simulink model "HANcoder_E407_TTA_Controller_v3_2"  (R2018b)
settings: Solver=FixedStepDiscrete  StartTime=0.0  StopTime=1  FixedStep=0.01  RelTol=1e-3
PreLoadFcn:
  | librarySetup
  | eval([bdroot,'_startup']) %Calling [modelName]_startup.m
undefined symbols (not defined in the file): A0, A1, A2, A3, A4, Backup_Board, basic_cycle_duration_bc0, basic_cycle_duration_bc1, comm_delay_estimation1, comm_delay_estimation2, COMM_Period, COMM_Phase1, COMM_Phase2, COMM_Phase_init1, COMM_Phase_init2, COMP_duration, CON2, CON4, Controller1_Board, Controller2_Board, Controller3_Board, D10, D12, D13, D8, D9, delta_a_set, delta_f_set, delta_max, delta_min, delta_precision, e_width, frequency_IRQ, HANtuneOverride, hardware_granularity, I_a, I_f, idle_time_init, Input_Gen_Board, LA_Clock_Gr, LA_COMM_dly, LA_COMM_Err, LA_E_Desync, LA_MEX_Flag, LA_Task_Act, m_v, Master_Role, matrix_cycle_duration, matrix_rows, max_desync, max_num_msgs_CAN1, max_num_msgs_CAN2, min_desync, OutControl1_ID, OutControl2_ID, OutEmulator_ID, R_al, R_ar, R_fl, R_fr ... (+80)
libraries: hdlsllib x434, HANcoder_STM32_Target x28, simulink x3, simulink_extras x1
(part 23 of 31)

== system HANcoder_E407_TTA_Controller_v3_2/HANcoder STM32 Target - E407-STM32 algorithm/TTA CAN System/TTA System/Matrix Cycle Manager/Vehicle Emulator Matrix Cycle/vehicle emulator basic cycle 1/COMM Task - Sync bc 1/Transmission subtasks/Check msg transmission CAN1 ==
  note: The TX buffers are updated one tick
      | before the message is sent
  note: A message should be sent during
      | this tick through CAN1
  note: In the next tick, a message will be
      | sent through CAN1
  Local Time : Inport
  Time Mark : Inport  Port=2
  Tx_ID : Inport  Port=3
  Value Domain Msg : Inport  Port=4
  Enable : EnablePort
  Constant : Constant  Value=COMM_Phase_init1
  Constant11 : Constant  Value=0
  Constant22 : Constant
  Constant24 : Constant  Value=COMM_Phase1
  Constant27 : Constant  Value=COMM_Phase1
  Constant8 : Constant  Value=0
  Equal4 : RelationalOperator  Operator===  OutDataTypeStr=boolean  RndMeth=Simplest
  Equal7 : RelationalOperator  Operator===  OutDataTypeStr=boolean  RndMeth=Simplest
  Minus : Sum  Inputs=++-
  Minus1 : Sum  Inputs=+-
  Minus2 : Sum
  Mod : Math  Operator=mod  SaturateOnIntegerOverflow=on
  Mod1 : Math  Operator=mod  SaturateOnIntegerOverflow=on
  TX buffer update CAN1 : Subsystem  Priority=20
  Send CAN1 : Outport  OutputWhenDisabled=reset  InitialOutput=0
  wires:
  Equal4/1 -> TX buffer update CAN1/Enable
  Constant22/1 -> Minus/2
  Local Time/1 -> Minus1/1, Minus/1
  Tx_ID/1 -> TX buffer update CAN1/1(Tx_ID)
  Mod1/1 -> Equal7/1
  Constant27/1 -> Mod1/2
  Minus/1 -> Mod/1
  Value Domain Msg/1 -> TX buffer update CAN1/2(Msg_Value_Data)
  Constant24/1 -> Mod/2
  Mod/1 -> Equal4/1
  Minus1/1 -> Mod1/1
  Constant11/1 -> Equal7/2
  Equal7/1 -> Send CAN1/1
  Constant8/1 -> Equal4/2
  Constant/1 -> Minus2/2
  Minus2/1 -> Minus1/2, Minus/3
  Time Mark/1 -> Minus2/1

== system HANcoder_E407_TTA_Controller_v3_2/HANcoder STM32 Target - E407-STM32 algorithm/TTA CAN System/TTA System/Matrix Cycle Manager/Vehicle Emulator Matrix Cycle/vehicle emulator basic cycle 1/COMM Task - Sync bc 1/Transmission subtasks/Check msg transmission CAN2 ==
  note: In the next tick, a message will be
      | sent through CAN2
  note: A message should be sent during
      | this tick through CAN2
  note: The TX buffers are updated one tick
      | before the message is sent
  Local Time : Inport
  Time Mark : Inport  Port=2
  Tx_ID : Inport  Port=3
  Value Domain Msg : Inport  Port=4
  Enable : EnablePort
  Constant : Constant  Value=COMM_Phase_init2
  Constant11 : Constant  Value=0
  Constant22 : Constant
  Constant24 : Constant  Value=COMM_Phase2
  Constant27 : Constant  Value=COMM_Phase2
  Constant8 : Constant  Value=0
  Equal4 : RelationalOperator  Operator===  OutDataTypeStr=boolean  RndMeth=Simplest
  Equal7 : RelationalOperator  Operator===  OutDataTypeStr=boolean  RndMeth=Simplest
  Minus : Sum  Inputs=++-
  Minus1 : Sum  Inputs=+-
  Minus2 : Sum
  Mod : Math  Operator=mod  SaturateOnIntegerOverflow=on
  Mod1 : Math  Operator=mod  SaturateOnIntegerOverflow=on
  TX buffer update CAN2 : Subsystem  Priority=20
  Send CAN2 : Outport  OutputWhenDisabled=reset  InitialOutput=0
  wires:
  Constant8/1 -> Equal4/2
  Equal7/1 -> Send CAN2/1
  Constant11/1 -> Equal7/2
  Minus1/1 -> Mod1/1
  Mod/1 -> Equal4/1
  Constant24/1 -> Mod/2
  Value Domain Msg/1 -> TX buffer update CAN2/2(Msg_Value_Data)
  Minus/1 -> Mod/1
  Constant27/1 -> Mod1/2
  Mod1/1 -> Equal7/1
  Tx_ID/1 -> TX buffer update CAN2/1(Tx_ID)
  Local Time/1 -> Minus/1, Minus1/1
  Constant22/1 -> Minus/2
  Equal4/1 -> TX buffer update CAN2/Enable
  Constant/1 -> Minus2/2
  Time Mark/1 -> Minus2/1
  Minus2/1 -> Minus1/2, Minus/3

== system HANcoder_E407_TTA_Controller_v3_2/HANcoder STM32 Target - E407-STM32 algorithm/TTA CAN System/TTA System/Matrix Cycle Manager/Vehicle Emulator Matrix Cycle/vehicle emulator basic cycle 1/COMM Task - Sync bc 1/Transmission subtasks/Msg_Value_Data_Encoded ==
  note: Value domain message encoding
      | <Warning!> The first buffer (from the top) is not used in transmission!
  Enable : EnablePort
  Bus Creator : BusCreator  Inputs=8  OutDataTypeStr=Bus: msg_buffer_type
  Constant : Constant  Value=0  OutDataTypeStr=uint8
  Constant1 : Constant  Value=torque_precision
  Constant10 : Constant  Value=speed_max
  Constant11 : Constant  Value=speed_min
  Constant12 : Constant  Value=delta_max
  Constant13 : Constant  Value=delta_min
  Constant14 : Constant  Value=delta_max
  Constant15 : Constant  Value=delta_min
  Constant2 : Constant  Value=torque_precision
  Constant3 : Constant  Value=speed_precision
  Constant4 : Constant  Value=delta_precision
  Constant5 : Constant  Value=delta_precision
  Constant6 : Constant  Value=tau_max
  Constant7 : Constant  Value=tau_min
  Constant8 : Constant  Value=tau_max
  Constant9 : Constant  Value=tau_min
  Data Store Read33 : DataStoreRead  DataStoreName=speed_integral
  Data Store Read34 : DataStoreRead  DataStoreName=torque_ar_integral
  Data Store Read35 : DataStoreRead  DataStoreName=torque_fr_integral
  Data Store Read36 : DataStoreRead  DataStoreName=delta_a_est
  Data Store Read37 : DataStoreRead  DataStoreName=delta_f_est
  float2uint1 : Subsystem
  float2uint2 : Subsystem
  float2uint3 : Subsystem
  float2uint4 : Subsystem
  float2uint8 : Subsystem
  Value_domain_msg : Outport
  wires:
  Bus Creator/1 -> Value_domain_msg/1
  Constant1/1 -> float2uint8/1(precision)
  Constant2/1 -> float2uint1/1(precision)
  Constant3/1 -> float2uint2/1(precision)
  Constant4/1 -> float2uint3/1(precision)
  Constant5/1 -> float2uint4/1(precision)
  Constant/1 -> Bus Creator/1, Bus Creator/8, Bus Creator/7
  Data Store Read35/1 -> float2uint8/2(magnitude)
  Data Store Read34/1 -> float2uint1/2(magnitude)
  Data Store Read33/1 -> float2uint2/2(magnitude)
  Data Store Read37/1 -> float2uint3/2(magnitude)
  Data Store Read36/1 -> float2uint4/2(magnitude)
  float2uint8/1(coded) -> Bus Creator/2
  float2uint1/1(coded) -> Bus Creator/3
  float2uint2/1(coded) -> Bus Creator/4
  float2uint3/1(coded) -> Bus Creator/5
  float2uint4/1(coded) -> Bus Creator/6
  Constant6/1 -> float2uint8/3(magnitude_max)
  Constant7/1 -> float2uint8/4(magnitude_min)
  Constant9/1 -> float2uint1/4(magnitude_min)
  Constant8/1 -> float2uint1/3(magnitude_max)
  Constant10/1 -> float2uint2/3(magnitude_max)
  Constant11/1 -> float2uint2/4(magnitude_min)
  Constant13/1 -> float2uint3/4(magnitude_min)
  Constant12/1 -> float2uint3/3(magnitude_max)
  Constant14/1 -> float2uint4/3(magnitude_max)
  Constant15/1 -> float2uint4/4(magnitude_min)

== system HANcoder_E407_TTA_Controller_v3_2/HANcoder STM32 Target - E407-STM32 algorithm/TTA CAN System/TTA System/Matrix Cycle Manager/Vehicle Emulator Matrix Cycle/vehicle emulator basic cycle 1/COMP Task - Rx Output Emulator Check/Process_Messages/Demux message CAN1 and check coherence ==
  CAN1_Rx_msg : Inport  OutDataTypeStr=Bus: msg_buffer_type
  expected_board_id : Inport  Port=2
  Enable : EnablePort
  Bus Creator : BusCreator  Inputs=8  OutDataTypeStr=Bus: msg_buffer_type
  Bus Selector : BusSelector  OutputSignals=Buffer_1,Buffer_2,Buffer_3,Buffer_4,Buffer_5,Buffer_6,Buffer_7,Buffer_8
  Constant : Constant  Value=0  OutDataTypeStr=uint8
  Equal : RelationalOperator  Operator===  OutDataTypeStr=boolean  RndMeth=Simplest
  Subsystem : Subsystem
  Terminator : Terminator
  msg_count>2_DEBUG : Subsystem
  CAN1_msg : Outport  OutDataTypeStr=Bus: msg_buffer_type
  Msg_Count_CAN1 : Outport  Port=2
  CAN1_msg_coherent : Outport  Port=3  OutputWhenDisabled=reset  InitialOutput=0
  wires:
  Bus Selector/2 -> Bus Creator/2  "<Buffer_2>"
  Bus Selector/3 -> Bus Creator/3  "<Buffer_3>"
  CAN1_Rx_msg/1 -> Bus Selector/1
  Equal/1 -> CAN1_msg_coherent/1
  expected_board_id/1 -> Equal/2
  Bus Selector/6 -> Bus Creator/6  "<Buffer_6>"
  Bus Selector/5 -> Bus Creator/5  "<Buffer_5>"
  Bus Selector/7 -> Bus Creator/7  "<Buffer_7>"
  Bus Selector/8 -> Bus Creator/8  "<Buffer_8>"
  Bus Selector/4 -> Bus Creator/4  "<Buffer_4>"
  Subsystem/3(board_id) -> Equal/1
  Bus Selector/1 -> Subsystem/1(Msg_Temporal_Data)  "<Buffer_1>"
  Subsystem/2(msg_count) -> msg_count>2_DEBUG/1(msg_c), Msg_Count_CAN1/1
  Bus Creator/1 -> CAN1_msg/1
  Constant/1 -> Bus Creator/1
  Subsystem/1(basic_cycle) -> Terminator/1

== system HANcoder_E407_TTA_Controller_v3_2/HANcoder STM32 Target - E407-STM32 algorithm/TTA CAN System/TTA System/Matrix Cycle Manager/Vehicle Emulator Matrix Cycle/vehicle emulator basic cycle 1/COMP Task - Rx Output Emulator Check/Process_Messages/Demux message CAN1 and check coherence1 ==
  CAN2_Rx_msg : Inport  OutDataTypeStr=Bus: msg_buffer_type
  expected_board_id : Inport  Port=2
  Enable : EnablePort
  Bus Creator : BusCreator  Inputs=8  OutDataTypeStr=Bus: msg_buffer_type
  Bus Selector : BusSelector  OutputSignals=Buffer_1,Buffer_2,Buffer_3,Buffer_4,Buffer_5,Buffer_6,Buffer_7,Buffer_8
  Constant : Constant  Value=0  OutDataTypeStr=uint8
  Equal : RelationalOperator  Operator===  OutDataTypeStr=boolean  RndMeth=Simplest
  Subsystem : Subsystem
  Terminator : Terminator
  msg_count>2_DEBUG : Subsystem
  CAN2_msg_coherent : Outport  OutputWhenDisabled=reset  InitialOutput=0
  Msg_Count_CAN2 : Outport  Port=2
  CAN2_msg : Outport  Port=3  OutDataTypeStr=Bus: msg_buffer_type
  wires:
  Bus Selector/2 -> Bus Creator/2  "<Buffer_2>"
  Bus Selector/3 -> Bus Creator/3  "<Buffer_3>"
  CAN2_Rx_msg/1 -> Bus Selector/1
  Equal/1 -> CAN2_msg_coherent/1
  expected_board_id/1 -> Equal/2
  Bus Selector/6 -> Bus Creator/6  "<Buffer_6>"
  Bus Selector/5 -> Bus Creator/5  "<Buffer_5>"
  Bus Selector/7 -> Bus Creator/7  "<Buffer_7>"
  Bus Selector/8 -> Bus Creator/8  "<Buffer_8>"
  Bus Selector/4 -> Bus Creator/4  "<Buffer_4>"
  Subsystem/3(board_id) -> Equal/1
  Bus Selector/1 -> Subsystem/1(Msg_Temporal_Data)  "<Buffer_1>"
  Subsystem/2(msg_count) -> msg_count>2_DEBUG/1(msg_c), Msg_Count_CAN2/1
  Bus Creator/1 -> CAN2_msg/1
  Constant/1 -> Bus Creator/1
  Subsystem/1(basic_cycle) -> Terminator/1

== system HANcoder_E407_TTA_Controller_v3_2/HANcoder STM32 Target - E407-STM32 algorithm/TTA CAN System/TTA System/Matrix Cycle Manager/Vehicle Emulator Matrix Cycle/vehicle emulator basic cycle 1/COMP Task - Rx Output Emulator Check/Update Msg buffer/Sensor Values Rx Update ==
  note: If we miss any msg, with current version we
      | suppose vehicle emulator remains in the same
      | state until new msg is received.
  note: Reinitialize variables
  note: Ticks to seconds conversion
  note: Matrix cycles since last input value
  note: For derivatives and integrals it is important to keep
      | track of how much time has passed since the last
      | time we received a controller value.
  msg_rx : Inport
  Enable : EnablePort
  Bus Selector : BusSelector  OutputSignals=Buffer_2,Buffer_3,Buffer_4,Buffer_5
  Constant : Constant  Value=matrix_cycle_duration
  Constant{1..4} (4 alike) : Constant  Value=torque_precision
  Constant5 : Constant
  Constant6 : Constant  Value=0  OutDataTypeStr=boolean
  Constant7 : Constant
  Data Store Read1 : DataStoreRead  DataStoreName=mc_counter
  Data Store Write : DataStoreWrite  DataStoreName=torque_fr
  Data Store Write1 : DataStoreWrite  DataStoreName=torque_fl
  Data Store Write2 : DataStoreWrite  DataStoreName=torque_ar
  Data Store Write3 : DataStoreWrite  DataStoreName=torque_al
  Data Store Write4 : DataStoreWrite  Priority=1  DataStoreName=rx_data_incr_time
  Data Store Write5 : DataStoreWrite  Priority=2  DataStoreName=mc_counter
  Data Store Write6 : DataStoreWrite  DataStoreName=controller_msg_missed
  Gain : Gain  Gain=frequency_IRQ/hardware_granularity
  Multiply : Product
  Terminator : Terminator
  uint8_2float : Subsystem
  uint8_2float1 : Subsystem
  uint8_2float2 : Subsystem
  uint8_2float3 : Subsystem
  wires:
  msg_rx/1 -> Bus Selector/1
  Bus Selector/3 -> uint8_2float2/2(value)  "<Buffer_4>"
  Bus Selector/2 -> uint8_2float1/2(value)  "<Buffer_3>"
  Bus Selector/1 -> uint8_2float/2(value)  "<Buffer_2>"
  Bus Selector/4 -> uint8_2float3/2(value)  "<Buffer_5>"
  Constant4/1 -> uint8_2float/1(precision)
  Constant1/1 -> uint8_2float1/1(precision)
  Constant2/1 -> uint8_2float2/1(precision)
  Constant3/1 -> uint8_2float3/1(precision)
  uint8_2float3/1(decoded) -> Data Store Write3/1
  uint8_2float2/1(decoded) -> Data Store Write2/1
  uint8_2float1/1(decoded) -> Data Store Write1/1
  uint8_2float/1(decoded) -> Data Store Write/1
  Constant5/1 -> Data Store Write5/1
  Gain/1 -> Multiply/1
  Constant7/1 -> Multiply/2
  Multiply/1 -> Data Store Write4/1
  Constant/1 -> Gain/1
  Constant6/1 -> Data Store Write6/1
  Data Store Read1/1 -> Terminator/1

== system HANcoder_E407_TTA_Controller_v3_2/HANcoder STM32 Target - E407-STM32 algorithm/TTA CAN System/TTA System/Matrix Cycle Manager/Vehicle Emulator Matrix Cycle/vehicle emulator basic cycle 1/COMP Task - Rx Output Emulator Check/Update Msg buffer/Sensor Values not Rx Update ==
  note: If no inputs received, no calculations are done.
      | Next time controller values are received
      | it is important to keep track of how much time
      | has passed for derivatives and integrals.
  Enable : EnablePort
  Constant1 : Constant
  Constant2 : Constant  OutDataTypeStr=boolean
  Data Store Read : DataStoreRead  DataStoreName=mc_counter
  Data Store Write : DataStoreWrite  DataStoreName=controller_msg_missed
  Data Store Write1 : DataStoreWrite  DataStoreName=mc_counter
  Minus : Sum
  wires:
  Minus/1 -> Data Store Write1/1
  Constant1/1 -> Minus/2
  Data Store Read/1 -> Minus/1
  Constant2/1 -> Data Store Write/1

== system HANcoder_E407_TTA_Controller_v3_2/HANcoder STM32 Target - E407-STM32 algorithm/TTA CAN System/TTA System/Matrix Cycle Manager/Vehicle Emulator Matrix Cycle/vehicle emulator basic cycle 1/COMP Task - Sync bc1 check/Process_Messages/Demux message CAN1 and check coherence ==
  CAN1_Rx_msg : Inport  OutDataTypeStr=Bus: msg_buffer_type
  expected_basic_cycle : Inport  Port=2
  Enable : EnablePort
  Bus Creator : BusCreator  Inputs=8  OutDataTypeStr=Bus: msg_buffer_type
  Bus Selector : BusSelector  OutputSignals=Buffer_1,Buffer_2,Buffer_3,Buffer_4,Buffer_5,Buffer_6,Buffer_7,Buffer_8
  Constant : Constant  Value=0  OutDataTypeStr=uint8
  Equal1 : RelationalOperator  Operator===  OutDataTypeStr=boolean  RndMeth=Simplest
  Subsystem : Subsystem
  Terminator : Terminator
  msg_count>2_DEBUG : Subsystem
  CAN1_msg : Outport  OutDataTypeStr=Bus: msg_buffer_type
  Msg_Count_CAN1 : Outport  Port=2
  CAN1_msg_coherent : Outport  Port=3  OutputWhenDisabled=reset  InitialOutput=0
  wires:
  Bus Selector/2 -> Bus Creator/2  "<Buffer_2>"
  Bus Selector/3 -> Bus Creator/3  "<Buffer_3>"
  CAN1_Rx_msg/1 -> Bus Selector/1
  Equal1/1 -> CAN1_msg_coherent/1
  expected_basic_cycle/1 -> Equal1/2
  Bus Selector/6 -> Bus Creator/6  "<Buffer_6>"
  Bus Selector/5 -> Bus Creator/5  "<Buffer_5>"
  Bus Selector/7 -> Bus Creator/7  "<Buffer_7>"
  Bus Selector/8 -> Bus Creator/8  "<Buffer_8>"
  Bus Selector/4 -> Bus Creator/4  "<Buffer_4>"
  Bus Selector/1 -> Subsystem/1(Msg_Temporal_Data)  "<Buffer_1>"
  Subsystem/1(basic_cycle) -> Equal1/1
  Subsystem/2(msg_count) -> msg_count>2_DEBUG/1(msg_c), Msg_Count_CAN1/1
  Bus Creator/1 -> CAN1_msg/1
  Constant/1 -> Bus Creator/1
  Subsystem/3(board_id) -> Terminator/1

== system HANcoder_E407_TTA_Controller_v3_2/HANcoder STM32 Target - E407-STM32 algorithm/TTA CAN System/TTA System/Matrix Cycle Manager/Vehicle Emulator Matrix Cycle/vehicle emulator basic cycle 1/COMP Task - Sync bc1 check/Process_Messages/Demux message CAN1 and check coherence1 ==
  CAN2_Rx_msg : Inport  OutDataTypeStr=Bus: msg_buffer_type
  expected_basic_cycle : Inport  Port=2
  Enable : EnablePort
  Bus Creator : BusCreator  Inputs=8  OutDataTypeStr=Bus: msg_buffer_type
  Bus Selector : BusSelector  OutputSignals=Buffer_1,Buffer_2,Buffer_3,Buffer_4,Buffer_5,Buffer_6,Buffer_7,Buffer_8
  Constant : Constant  Value=0  OutDataTypeStr=uint8
  Equal1 : RelationalOperator  Operator===  OutDataTypeStr=boolean  RndMeth=Simplest
  Subsystem : Subsystem
  Terminator : Terminator
  msg_count>2_DEBUG : Subsystem
  CAN2_msg_coherent : Outport  OutputWhenDisabled=reset  InitialOutput=0
  Msg_Count_CAN2 : Outport  Port=2
  CAN2_msg : Outport  Port=3  OutDataTypeStr=Bus: msg_buffer_type
  wires:
  Bus Selector/2 -> Bus Creator/2  "<Buffer_2>"
  Bus Selector/3 -> Bus Creator/3  "<Buffer_3>"
  CAN2_Rx_msg/1 -> Bus Selector/1
  Equal1/1 -> CAN2_msg_coherent/1
  expected_basic_cycle/1 -> Equal1/2
  Bus Selector/6 -> Bus Creator/6  "<Buffer_6>"
  Bus Selector/5 -> Bus Creator/5  "<Buffer_5>"
  Bus Selector/7 -> Bus Creator/7  "<Buffer_7>"
  Bus Selector/8 -> Bus Creator/8  "<Buffer_8>"
  Bus Selector/4 -> Bus Creator/4  "<Buffer_4>"
  Bus Selector/1 -> Subsystem/1(Msg_Temporal_Data)  "<Buffer_1>"
  Subsystem/1(basic_cycle) -> Equal1/1
  Subsystem/2(msg_count) -> Msg_Count_CAN2/1, msg_count>2_DEBUG/1(msg_c)
  Bus Creator/1 -> CAN2_msg/1
  Constant/1 -> Bus Creator/1
  Subsystem/3(board_id) -> Terminator/1

== system HANcoder_E407_TTA_Controller_v3_2/HANcoder STM32 Target - E407-STM32 algorithm/TTA CAN System/TTA System/Matrix Cycle Manager/Vehicle Emulator Matrix Cycle/vehicle emulator basic cycle 1/COMP Task - Sync bc1 check/Process_Messages/Desync calculation ==
  note: Estimation of the Local Time when the message was sent
  note: Desync CAN2
      | expected RX - Actual RX
  note: Desync CAN1
      | expected RX - Actual RX
  TM_COMM : Inport
  New_msg_CAN1 : Inport  Port=2
  msg_count_CAN1 : Inport  Port=3
  msg_count_CAN2 : Inport  Port=4
  Enable : EnablePort
  Constant : Constant  Value=COMM_Phase1
  Constant1 : Constant  Value=COMM_Phase2
  Data Store Read : DataStoreRead  DataStoreName=Msg_Rx_Ticks_CAN1
  Data Store Read1 : DataStoreRead  DataStoreName=Msg_Rx_Ticks_CAN2
  Data Store Write1 : DataStoreWrite  Priority=23  DataStoreName=Desync_Ticks
  Minus : Sum  Priority=21  Inputs=+-
  Minus1 : Sum  Priority=20  Inputs=+-
  Multiply : Product  Priority=10
  Multiply1 : Product  Priority=12
  Saturation : Saturate  UpperLimit=max_desync  LowerLimit=min_desync
  Sum : Sum  Priority=11  Inputs=+++
  Sum1 : Sum  Priority=13  Inputs=+++
  Switch1 : Switch  Priority=22  Criteria=u2 > Threshold
  delay_estimation_1 : Constant  Value=comm_delay_estimation1
  delay_estimation_2 : Constant  Value=comm_delay_estimation2
  wires:
  TM_COMM/1 -> Sum1/2, Sum/2
  delay_estimation_1/1 -> Sum/3
  msg_count_CAN1/1 -> Multiply/2
  Switch1/1 -> Saturation/1
  Minus/1 -> Switch1/3
  Sum1/1 -> [expected_LT_CAN2]
  delay_estimation_2/1 -> Sum1/3
  Multiply1/1 -> Sum1/1
  [expected_LT_CAN1] -> Minus1/1
  [expected_LT_CAN2] -> Minus/1
  Data Store Read1/1 -> Minus/2
  Multiply/1 -> Sum/1
  Data Store Read/1 -> Minus1/2
  msg_count_CAN2/1 -> Multiply1/2
  Sum/1 -> [expected_LT_CAN1]
  Minus1/1 -> Switch1/1
  Constant/1 -> Multiply/1
  Constant1/1 -> Multiply1/1
  New_msg_CAN1/1 -> Switch1/2
  Saturation/1 -> Data Store Write1/1  "Desync_Sync_bc1_vem_s"

== system HANcoder_E407_TTA_Controller_v3_2/HANcoder STM32 Target - E407-STM32 algorithm/TTA CAN System/TTA System/Matrix Cycle Manager/Vehicle Emulator Matrix Cycle/vehicle emulator basic cycle 1/COMP Task - Update LT/Local Time Update/Desync_Negative ==
  note: Local Time Update
  note: Current Local Time correction
  note: Local time correction when Desync is negative
      | In this case the Local Time "goes back in time".
      | Previous tasks will not be activated because
      | sync_processed flag is alread set.
  Current_Local_Time : Inport
  Enable : EnablePort
  Cast : DataTypeConversion  Priority=13  OutDataTypeStr=uint16
  Data Store Read : DataStoreRead  Priority=11  DataStoreName=Desync_Ticks
  Data Store Write1 : DataStoreWrite  Priority=14  DataStoreName=Local_Ticks  DataStoreElements=Local_Ticks
  Minus : Sum  Priority=12
  wires:
  Current_Local_Time/1 -> Minus/1
  Cast/1 -> Data Store Write1/1
  Minus/1 -> Cast/1
  Data Store Read/1 -> Minus/2

== system HANcoder_E407_TTA_Controller_v3_2/HANcoder STM32 Target - E407-STM32 algorithm/TTA CAN System/TTA System/Matrix Cycle Manager/Backup Board Matrix Cycle/Backup board basic cycle 0/COMM Task - Sync bc 0/Transmission subtasks/Check msg transmission CAN1/TX buffer update CAN1 ==
  note: Transmission end - Set message to send through CAN 1
  note: Message Temporal Data
      |    Every message sends
      |    BasicCycle, Tx count
      |    and Verification msg
      |    as data
  note: Transmission ID
      |    Sync Msg: 1
      |    Vote Node 1: 11
      |    Vote Node 2: 12
      |    Vote Node 3: 13
  Tx_ID : Inport
  Msg_Value_Data : Inport  Port=2
  Enable : EnablePort
  Bus Selector : BusSelector  OutputSignals=signal2,signal3,signal4,signal5,signal6,signal7,signal8
  Cast : DataTypeConversion  OutDataTypeStr=uint32
  Cast1 : DataTypeConversion  OutDataTypeStr=uint8
  Cast16 : DataTypeConversion  OutDataTypeStr=uint8
  Cast4 : DataTypeConversion  OutDataTypeStr=uint8
  Data Store Read : DataStoreRead  Priority=50  DataStoreName=Tx_msg_count_CAN1
  Data Store Read1 : DataStoreRead  DataStoreName=Board_ID
  Data Store Read3 : DataStoreRead  DataStoreName=basic_cycle_count
  Data Store Write10 : DataStoreWrite  DataStoreName=Msg_Tx_CAN1  DataStoreElements=Msg_Tx_CAN1.Buffer_1#Msg_Tx_CAN1.Buffer_2#Msg_Tx_CAN1.Buffer_3#Msg_Tx_CAN1.Buffer_4#Msg_Tx_CAN1.Buffer_5#Msg_Tx_CAN1.Buffer_6#Msg_Tx_CAN1.Buffer_7#Msg_Tx_CAN1.Buffer_8
  Data Store Write8 : DataStoreWrite  DataStoreName=TxID_CAN1
  Msg_Data_Encoder : Subsystem
  wires:
  Cast/1 -> Data Store Write8/1
  Data Store Read3/1 -> Cast4/1
  Cast4/1 -> Msg_Data_Encoder/1(basic_cycle)
  Msg_Value_Data/1 -> Bus Selector/1
  Tx_ID/1 -> Cast/1
  Data Store Read/1 -> Cast1/1
  Cast16/1 -> Msg_Data_Encoder/3(board_number)
  Cast1/1 -> Msg_Data_Encoder/2(tx_counter)
  Data Store Read1/1 -> Cast16/1
  Msg_Data_Encoder/1(encoded_msg) -> Data Store Write10/1
  Bus Selector/1 -> Data Store Write10/2  "<signal2>"
  Bus Selector/2 -> Data Store Write10/3  "<signal3>"
  Bus Selector/3 -> Data Store Write10/4  "<signal4>"
  Bus Selector/4 -> Data Store Write10/5  "<signal5>"
  Bus Selector/5 -> Data Store Write10/6  "<signal6>"
  Bus Selector/6 -> Data Store Write10/7  "<signal7>"
  Bus Selector/7 -> Data Store Write10/8  "<signal8>"

== system HANcoder_E407_TTA_Controller_v3_2/HANcoder STM32 Target - E407-STM32 algorithm/TTA CAN System/TTA System/Matrix Cycle Manager/Backup Board Matrix Cycle/Backup board basic cycle 0/COMM Task - Sync bc 0/Transmission subtasks/Check msg transmission CAN2/TX buffer update CAN2 ==
  note: Transmission end - Set message to send through CAN
  note: Transmission ID
      |    Sync Msg: 1
      |    Vote Node 1: 11
      |    Vote Node 2: 12
      |    Vote Node 3: 13
  note: Message Data
      |    Every message sends
      |    BasicCycle, Tx count
      |    and Verification msg
      |    as data
  Tx_ID : Inport
  Msg_Value_Data : Inport  Port=2
  Enable : EnablePort
  Bus Selector : BusSelector  OutputSignals=signal2,signal3,signal4,signal5,signal6,signal7,signal8
  Cast17 : DataTypeConversion  OutDataTypeStr=uint8
  Cast18 : DataTypeConversion  OutDataTypeStr=uint8
  Cast8 : DataTypeConversion  OutDataTypeStr=uint32
  Cast9 : DataTypeConversion  OutDataTypeStr=uint8
  Data Store Read : DataStoreRead  DataStoreName=Board_ID
  Data Store Read1 : DataStoreRead  Priority=50  DataStoreName=Tx_msg_count_CAN2
  Data Store Read6 : DataStoreRead  DataStoreName=basic_cycle_count
  Data Store Write4 : DataStoreWrite  DataStoreName=Msg_Tx_CAN2  DataStoreElements=Msg_Tx_CAN2.Buffer_1#Msg_Tx_CAN2.Buffer_2#Msg_Tx_CAN2.Buffer_3#Msg_Tx_CAN2.Buffer_4#Msg_Tx_CAN2.Buffer_5#Msg_Tx_CAN2.Buffer_6#Msg_Tx_CAN2.Buffer_7#Msg_Tx_CAN2.Buffer_8
  Data Store Write5 : DataStoreWrite  DataStoreName=TxID_CAN2
  Msg_Data_Encoder : Subsystem
  wires:
  Bus Selector/7 -> Data Store Write4/8  "<signal8>"
  Bus Selector/6 -> Data Store Write4/7  "<signal7>"
  Bus Selector/5 -> Data Store Write4/6  "<signal6>"
  Bus Selector/4 -> Data Store Write4/5  "<signal5>"
  Bus Selector/3 -> Data Store Write4/4  "<signal4>"
  Bus Selector/2 -> Data Store Write4/3  "<signal3>"
  Bus Selector/1 -> Data Store Write4/2  "<signal2>"
  Msg_Value_Data/1 -> Bus Selector/1
  Data Store Read/1 -> Cast17/1
  Cast8/1 -> Data Store Write5/1
  Cast9/1 -> Msg_Data_Encoder/2(tx_counter)
  Tx_ID/1 -> Cast8/1
  Cast17/1 -> Msg_Data_Encoder/3(verif_value)
  Data Store Read6/1 -> Cast18/1
  Msg_Data_Encoder/1(encoded_msg) -> Data Store Write4/1
  Data Store Read1/1 -> Cast9/1
  Cast18/1 -> Msg_Data_Encoder/1(basic_cycle)

== system HANcoder_E407_TTA_Controller_v3_2/HANcoder STM32 Target - E407-STM32 algorithm/TTA CAN System/TTA System/Matrix Cycle Manager/Backup Board Matrix Cycle/Backup board basic cycle 0/COMM Task - Sync bc 0/Transmission subtasks/Msg_Value_Data_Encoded/float2uint1 ==
  precision : Inport
  magnitude : Inport  Port=2
  magnitude_max : Inport  Port=3
  magnitude_min : Inport  Port=4
  Abs : Abs
  Bit Shift : hdlsllib/Logic and Bit Operations/Bit Shift  mode=Shift Left Logical  N=7
      settings: SourceProductName=HDL Coder  SourceProductBaseCode=HD
  Cast : DataTypeConversion  OutDataTypeStr=uint8
  Cast1 : DataTypeConversion  OutDataTypeStr=uint8
  Cast2 : DataTypeConversion  OutDataTypeStr=uint8
  Constant : Constant  Value=0
  Constant1 : Constant  Value=2
  Constant2 : Constant  Value=2
  Divide : Product  Inputs=*/
  Fix : Rounding  Priority=3  Operator=fix
  Fix1 : Rounding  Priority=6  Operator=fix
  Gain : Gain  Gain=-1
  GreaterThan : RelationalOperator  Priority=2  Operator=<  OutDataTypeStr=boolean  RndMeth=Simplest
  LessThanOrEqual1 : RelationalOperator  OutDataTypeStr=boolean  RndMeth=Simplest
  LessThanOrEqual2 : RelationalOperator  Operator=<  OutDataTypeStr=boolean  RndMeth=Simplest
  Minus : Sum  Priority=4  Inputs=-+
  Multiply : Product
  Plus : Sum  Priority=10  Inputs=+++
  Power : Math  Priority=5  Operator=pow  SaturateOnIntegerOverflow=on
  Power1 : Math  Priority=5  Operator=pow  SaturateOnIntegerOverflow=on
  Switch : Switch  Criteria=u2 > Threshold
  Switch1 : Switch  Criteria=u2 > Threshold
  Switch2 : Switch  Criteria=u2 > Threshold
  coded : Outport
  wires:
  Switch1/1 -> Switch2/3
  Switch/1 -> Switch2/1
  LessThanOrEqual1/1 -> Switch1/2
  LessThanOrEqual2/1 -> Switch/2, Switch2/2
  magnitude_max/1 -> LessThanOrEqual2/1, Switch/1
  magnitude_min/1 -> Switch1/3, LessThanOrEqual1/2
  magnitude/1 -> Switch/3, LessThanOrEqual2/2, Switch1/1, LessThanOrEqual1/1
  Plus/1 -> coded/1
  [prec] -> Power1/2
  Multiply/1 -> Cast1/1
  precision/1 -> Gain/1, [prec]
  Power1/1 -> Multiply/2
  Constant2/1 -> Power1/1
  Cast2/1 -> Plus/3
  Fix1/1 -> Cast2/1
  Divide/1 -> Fix1/1
  Power/1 -> Divide/2
  Gain/1 -> Power/2
  Constant1/1 -> Power/1
  Cast1/1 -> Plus/2
  Bit Shift/1 -> Plus/1
  Cast/1 -> Bit Shift/1
  Minus/1 -> Divide/1
  Fix/1 -> Minus/1, Multiply/1
  GreaterThan/1 -> Cast/1
  Abs/1 -> Fix/1, Minus/2
  Switch2/1 -> GreaterThan/1, Abs/1
  Constant/1 -> GreaterThan/2

== system HANcoder_E407_TTA_Controller_v3_2/HANcoder STM32 Target - E407-STM32 algorithm/TTA CAN System/TTA System/Matrix Cycle Manager/Backup Board Matrix Cycle/Backup board basic cycle 0/COMM Task - Sync bc 0/Transmission subtasks/Msg_Value_Data_Encoded/float2uint2 ==
  precision : Inport
  magnitude : Inport  Port=2
  magnitude_max : Inport  Port=3
  magnitude_min : Inport  Port=4
  Abs : Abs
  Bit Shift : hdlsllib/Logic and Bit Operations/Bit Shift  mode=Shift Left Logical  N=7
      settings: SourceProductName=HDL Coder  SourceProductBaseCode=HD
  Cast : DataTypeConversion  OutDataTypeStr=uint8
  Cast1 : DataTypeConversion  OutDataTypeStr=uint8
  Cast2 : DataTypeConversion  OutDataTypeStr=uint8
  Constant : Constant  Value=0
  Constant1 : Constant  Value=2
  Constant2 : Constant  Value=2
  Divide : Product  Inputs=*/
  Fix : Rounding  Priority=3  Operator=fix
  Fix1 : Rounding  Priority=6  Operator=fix
  Gain : Gain  Gain=-1
  GreaterThan : RelationalOperator  Priority=2  Operator=<  OutDataTypeStr=boolean  RndMeth=Simplest
  LessThanOrEqual1 : RelationalOperator  OutDataTypeStr=boolean  RndMeth=Simplest
  LessThanOrEqual2 : RelationalOperator  Operator=<  OutDataTypeStr=boolean  RndMeth=Simplest
  Minus : Sum  Priority=4  Inputs=-+
  Multiply : Product
  Plus : Sum  Priority=10  Inputs=+++
  Power : Math  Priority=5  Operator=pow  SaturateOnIntegerOverflow=on
  Power1 : Math  Priority=5  Operator=pow  SaturateOnIntegerOverflow=on
  Switch : Switch  Criteria=u2 > Threshold
  Switch1 : Switch  Criteria=u2 > Threshold
  Switch2 : Switch  Criteria=u2 > Threshold
  coded : Outport
  wires:
  Constant/1 -> GreaterThan/2
  Switch2/1 -> Abs/1, GreaterThan/1
  Abs/1 -> Minus/2, Fix/1
  GreaterThan/1 -> Cast/1
  Fix/1 -> Multiply/1, Minus/1
  Minus/1 -> Divide/1
  Cast/1 -> Bit Shift/1
  Bit Shift/1 -> Plus/1
  Cast1/1 -> Plus/2
  Constant1/1 -> Power/1
  Gain/1 -> Power/2
  Power/1 -> Divide/2
  Divide/1 -> Fix1/1
  Fix1/1 -> Cast2/1
  Cast2/1 -> Plus/3
  Constant2/1 -> Power1/1
  Power1/1 -> Multiply/2
  precision/1 -> [prec], Gain/1
  Multiply/1 -> Cast1/1
  [prec] -> Power1/2
  Plus/1 -> coded/1
  magnitude/1 -> LessThanOrEqual1/1, Switch1/1, LessThanOrEqual2/2, Switch/3
  magnitude_min/1 -> LessThanOrEqual1/2, Switch1/3
  magnitude_max/1 -> Switch/1, LessThanOrEqual2/1
  LessThanOrEqual2/1 -> Switch2/2, Switch/2
  LessThanOrEqual1/1 -> Switch1/2
  Switch/1 -> Switch2/1
  Switch1/1 -> Switch2/3

== system HANcoder_E407_TTA_Controller_v3_2/HANcoder STM32 Target - E407-STM32 algorithm/TTA CAN System/TTA System/Matrix Cycle Manager/Backup Board Matrix Cycle/Backup board basic cycle 0/COMM Task - Sync bc 0/Transmission subtasks/Msg_Value_Data_Encoded/float2uint3 ==
  precision : Inport
  magnitude : Inport  Port=2
  magnitude_max : Inport  Port=3
  magnitude_min : Inport  Port=4
  Abs : Abs
  Bit Shift : hdlsllib/Logic and Bit Operations/Bit Shift  mode=Shift Left Logical  N=7
      settings: SourceProductName=HDL Coder  SourceProductBaseCode=HD
  Cast : DataTypeConversion  OutDataTypeStr=uint8
  Cast1 : DataTypeConversion  OutDataTypeStr=uint8
  Cast2 : DataTypeConversion  OutDataTypeStr=uint8
  Constant : Constant  Value=0
  Constant1 : Constant  Value=2
  Constant2 : Constant  Value=2
  Divide : Product  Inputs=*/
  Fix : Rounding  Priority=3  Operator=fix
  Fix1 : Rounding  Priority=6  Operator=fix
  Gain : Gain  Gain=-1
  GreaterThan : RelationalOperator  Priority=2  Operator=<  OutDataTypeStr=boolean  RndMeth=Simplest
  LessThanOrEqual1 : RelationalOperator  OutDataTypeStr=boolean  RndMeth=Simplest
  LessThanOrEqual2 : RelationalOperator  Operator=<  OutDataTypeStr=boolean  RndMeth=Simplest
  Minus : Sum  Priority=4  Inputs=-+
  Multiply : Product
  Plus : Sum  Priority=10  Inputs=+++
  Power : Math  Priority=5  Operator=pow  SaturateOnIntegerOverflow=on
  Power1 : Math  Priority=5  Operator=pow  SaturateOnIntegerOverflow=on
  Switch : Switch  Criteria=u2 > Threshold
  Switch1 : Switch  Criteria=u2 > Threshold
  Switch2 : Switch  Criteria=u2 > Threshold
  coded : Outport
  wires:
  Switch1/1 -> Switch2/3
  Switch/1 -> Switch2/1
  LessThanOrEqual1/1 -> Switch1/2
  LessThanOrEqual2/1 -> Switch/2, Switch2/2
  magnitude_max/1 -> LessThanOrEqual2/1, Switch/1
  magnitude_min/1 -> Switch1/3, LessThanOrEqual1/2
  magnitude/1 -> Switch/3, LessThanOrEqual2/2, Switch1/1, LessThanOrEqual1/1
  Plus/1 -> coded/1
  [prec] -> Power1/2
  Multiply/1 -> Cast1/1
  precision/1 -> Gain/1, [prec]
  Power1/1 -> Multiply/2
  Constant2/1 -> Power1/1
  Cast2/1 -> Plus/3
  Fix1/1 -> Cast2/1
  Divide/1 -> Fix1/1
  Power/1 -> Divide/2
  Gain/1 -> Power/2
  Constant1/1 -> Power/1
  Cast1/1 -> Plus/2
  Bit Shift/1 -> Plus/1
  Cast/1 -> Bit Shift/1
  Minus/1 -> Divide/1
  Fix/1 -> Minus/1, Multiply/1
  GreaterThan/1 -> Cast/1
  Abs/1 -> Fix/1, Minus/2
  Switch2/1 -> GreaterThan/1, Abs/1
  Constant/1 -> GreaterThan/2

== system HANcoder_E407_TTA_Controller_v3_2/HANcoder STM32 Target - E407-STM32 algorithm/TTA CAN System/TTA System/Matrix Cycle Manager/Backup Board Matrix Cycle/Backup board basic cycle 0/COMM Task - Sync bc 0/Transmission subtasks/Msg_Value_Data_Encoded/float2uint4 ==
  precision : Inport
  magnitude : Inport  Port=2
  magnitude_max : Inport  Port=3
  magnitude_min : Inport  Port=4
  Abs : Abs
  Bit Shift : hdlsllib/Logic and Bit Operations/Bit Shift  mode=Shift Left Logical  N=7
      settings: SourceProductName=HDL Coder  SourceProductBaseCode=HD
  Cast : DataTypeConversion  OutDataTypeStr=uint8
  Cast1 : DataTypeConversion  OutDataTypeStr=uint8
  Cast2 : DataTypeConversion  OutDataTypeStr=uint8
  Constant : Constant  Value=0
  Constant1 : Constant  Value=2
  Constant2 : Constant  Value=2
  Divide : Product  Inputs=*/
  Fix : Rounding  Priority=3  Operator=fix
  Fix1 : Rounding  Priority=6  Operator=fix
  Gain : Gain  Gain=-1
  GreaterThan : RelationalOperator  Priority=2  Operator=<  OutDataTypeStr=boolean  RndMeth=Simplest
  LessThanOrEqual1 : RelationalOperator  OutDataTypeStr=boolean  RndMeth=Simplest
  LessThanOrEqual2 : RelationalOperator  Operator=<  OutDataTypeStr=boolean  RndMeth=Simplest
  Minus : Sum  Priority=4  Inputs=-+
  Multiply : Product
  Plus : Sum  Priority=10  Inputs=+++
  Power : Math  Priority=5  Operator=pow  SaturateOnIntegerOverflow=on
  Power1 : Math  Priority=5  Operator=pow  SaturateOnIntegerOverflow=on
  Switch : Switch  Criteria=u2 > Threshold
  Switch1 : Switch  Criteria=u2 > Threshold
  Switch2 : Switch  Criteria=u2 > Threshold
  coded : Outport
  wires:
  Constant/1 -> GreaterThan/2
  Switch2/1 -> Abs/1, GreaterThan/1
  Abs/1 -> Minus/2, Fix/1
  GreaterThan/1 -> Cast/1
  Fix/1 -> Multiply/1, Minus/1
  Minus/1 -> Divide/1
  Cast/1 -> Bit Shift/1
  Bit Shift/1 -> Plus/1
  Cast1/1 -> Plus/2
  Constant1/1 -> Power/1
  Gain/1 -> Power/2
  Power/1 -> Divide/2
  Divide/1 -> Fix1/1
  Fix1/1 -> Cast2/1
  Cast2/1 -> Plus/3
  Constant2/1 -> Power1/1
  Power1/1 -> Multiply/2
  precision/1 -> [prec], Gain/1
  Multiply/1 -> Cast1/1
  [prec] -> Power1/2
  Plus/1 -> coded/1
  magnitude/1 -> LessThanOrEqual1/1, Switch1/1, LessThanOrEqual2/2, Switch/3
  magnitude_min/1 -> LessThanOrEqual1/2, Switch1/3
  magnitude_max/1 -> Switch/1, LessThanOrEqual2/1
  LessThanOrEqual2/1 -> Switch2/2, Switch/2
  LessThanOrEqual1/1 -> Switch1/2
  Switch/1 -> Switch2/1
  Switch1/1 -> Switch2/3

== system HANcoder_E407_TTA_Controller_v3_2/HANcoder STM32 Target - E407-STM32 algorithm/TTA CAN System/TTA System/Matrix Cycle Manager/Backup Board Matrix Cycle/Backup board basic cycle 0/COMM Task - Sync bc 0/Transmission subtasks/Msg_Value_Data_Encoded/float2uint8 ==
  precision : Inport
  magnitude : Inport  Port=2
  magnitude_max : Inport  Port=3
  magnitude_min : Inport  Port=4
  Abs : Abs
  Bit Shift : hdlsllib/Logic and Bit Operations/Bit Shift  mode=Shift Left Logical  N=7
      settings: SourceProductName=HDL Coder  SourceProductBaseCode=HD
  Cast : DataTypeConversion  OutDataTypeStr=uint8
  Cast1 : DataTypeConversion  OutDataTypeStr=uint8
  Cast2 : DataTypeConversion  OutDataTypeStr=uint8
  Constant : Constant  Value=0
  Constant1 : Constant  Value=2
  Constant2 : Constant  Value=2
  Divide : Product  Inputs=*/
  Fix : Rounding  Priority=3  Operator=fix
  Fix1 : Rounding  Priority=6  Operator=fix
  Gain : Gain  Gain=-1
  GreaterThan : RelationalOperator  Priority=2  Operator=<  OutDataTypeStr=boolean  RndMeth=Simplest
  LessThanOrEqual1 : RelationalOperator  OutDataTypeStr=boolean  RndMeth=Simplest
  LessThanOrEqual2 : RelationalOperator  Operator=<  OutDataTypeStr=boolean  RndMeth=Simplest
  Minus : Sum  Priority=4  Inputs=-+
  Multiply : Product
  Plus : Sum  Priority=10  Inputs=+++
  Power : Math  Priority=5  Operator=pow  SaturateOnIntegerOverflow=on
  Power1 : Math  Priority=5  Operator=pow  SaturateOnIntegerOverflow=on
  Switch : Switch  Criteria=u2 > Threshold
  Switch1 : Switch  Criteria=u2 > Threshold
  Switch2 : Switch  Criteria=u2 > Threshold
  coded : Outport
  wires:
  Constant/1 -> GreaterThan/2
  Switch2/1 -> Abs/1, GreaterThan/1
  Abs/1 -> Minus/2, Fix/1
  GreaterThan/1 -> Cast/1
  Fix/1 -> Multiply/1, Minus/1
  Minus/1 -> Divide/1
  Cast/1 -> Bit Shift/1
  Bit Shift/1 -> Plus/1
  Cast1/1 -> Plus/2
  Constant1/1 -> Power/1
  Gain/1 -> Power/2
  Power/1 -> Divide/2
  Divide/1 -> Fix1/1
  Fix1/1 -> Cast2/1
  Cast2/1 -> Plus/3
  Constant2/1 -> Power1/1
  Power1/1 -> Multiply/2
  precision/1 -> [prec], Gain/1
  Multiply/1 -> Cast1/1
  [prec] -> Power1/2
  Plus/1 -> coded/1
  magnitude/1 -> LessThanOrEqual1/1, Switch1/1, LessThanOrEqual2/2, Switch/3
  magnitude_min/1 -> LessThanOrEqual1/2, Switch1/3
  magnitude_max/1 -> Switch/1, LessThanOrEqual2/1
  LessThanOrEqual2/1 -> Switch2/2, Switch/2
  LessThanOrEqual1/1 -> Switch1/2
  Switch/1 -> Switch2/1
  Switch1/1 -> Switch2/3

== system HANcoder_E407_TTA_Controller_v3_2/HANcoder STM32 Target - E407-STM32 algorithm/TTA CAN System/TTA System/Matrix Cycle Manager/Backup Board Matrix Cycle/Backup board basic cycle 0/COMP Task - Sync bc0 check/Process_Messages/Demux message CAN1 and check coherence/Subsystem ==
  Msg_Temporal_Data : Inport
  Bit Shift : hdlsllib/Logic and Bit Operations/Bit Shift  mode=Shift Right Logical  N=7
      settings: SourceProductName=HDL Coder  SourceProductBaseCode=HD
  Bit Shift1 : hdlsllib/Logic and Bit Operations/Bit Shift  mode=Shift Right Logical  N=5
      settings: SourceProductName=HDL Coder  SourceProductBaseCode=HD
  Bit Shift2 : hdlsllib/Logic and Bit Operations/Bit Shift  mode=Shift Right Logical  N=4
      settings: SourceProductName=HDL Coder  SourceProductBaseCode=HD
  Bit Shift3 : hdlsllib/Logic and Bit Operations/Bit Shift  mode=Shift Left Logical  N=1
      settings: SourceProductName=HDL Coder  SourceProductBaseCode=HD
  Bit Shift4 : hdlsllib/Logic and Bit Operations/Bit Shift  mode=Shift Left Logical  N=4
      settings: SourceProductName=HDL Coder  SourceProductBaseCode=HD
  basic_cycle : Outport
  msg_count : Outport  Port=2
  board_id : Outport  Port=3
  wires:
  Bit Shift4/1 -> Bit Shift2/1
  Bit Shift1/1 -> msg_count/1
  Bit Shift3/1 -> Bit Shift1/1
  Msg_Temporal_Data/1 -> Bit Shift4/1, Bit Shift/1, Bit Shift3/1
  Bit Shift/1 -> basic_cycle/1
  Bit Shift2/1 -> board_id/1

== system HANcoder_E407_TTA_Controller_v3_2/HANcoder STM32 Target - E407-STM32 algorithm/TTA CAN System/TTA System/Matrix Cycle Manager/Backup Board Matrix Cycle/Backup board basic cycle 0/COMP Task - Sync bc0 check/Process_Messages/Demux message CAN1 and check coherence/msg_count>2_DEBUG ==
  note: If this board received during this COMM a message
      | with a count greater than 1, it means the first message
      | sent was missed, but at least one later msg reached
      | this board.
  msg_c : Inport
  Constant : Constant
  Constant1 : Constant
  Data Store Read : DataStoreRead  DataStoreName=msg_count_DEBUG
  Data Store Read1 : DataStoreRead  DataStoreName=msg_count_DEBUG
  Data Store Write : DataStoreWrite  DataStoreName=msg_count_DEBUG
  GreaterThan : RelationalOperator  Operator=>  OutDataTypeStr=boolean  RndMeth=Simplest
  Plus : Sum
  Switch : Switch  Criteria=u2 > Threshold
  wires:
  msg_c/1 -> GreaterThan/1
  Data Store Read/1 -> Switch/3
  Plus/1 -> Switch/1
  Data Store Read1/1 -> Plus/1
  Constant/1 -> Plus/2
  Switch/1 -> Data Store Write/1
  GreaterThan/1 -> Switch/2
  Constant1/1 -> GreaterThan/2

== system HANcoder_E407_TTA_Controller_v3_2/HANcoder STM32 Target - E407-STM32 algorithm/TTA CAN System/TTA System/Matrix Cycle Manager/Backup Board Matrix Cycle/Backup board basic cycle 0/COMP Task - Sync bc0 check/Process_Messages/Demux message CAN1 and check coherence1/Subsystem ==
  Msg_Temporal_Data : Inport
  Bit Shift : hdlsllib/Logic and Bit Operations/Bit Shift  mode=Shift Right Logical  N=7
      settings: SourceProductName=HDL Coder  SourceProductBaseCode=HD
  Bit Shift1 : hdlsllib/Logic and Bit Operations/Bit Shift  mode=Shift Right Logical  N=5
      settings: SourceProductName=HDL Coder  SourceProductBaseCode=HD
  Bit Shift2 : hdlsllib/Logic and Bit Operations/Bit Shift  mode=Shift Right Logical  N=4
      settings: SourceProductName=HDL Coder  SourceProductBaseCode=HD
  Bit Shift3 : hdlsllib/Logic and Bit Operations/Bit Shift  mode=Shift Left Logical  N=1
      settings: SourceProductName=HDL Coder  SourceProductBaseCode=HD
  Bit Shift4 : hdlsllib/Logic and Bit Operations/Bit Shift  mode=Shift Left Logical  N=4
      settings: SourceProductName=HDL Coder  SourceProductBaseCode=HD
  basic_cycle : Outport
  msg_count : Outport  Port=2
  board_id : Outport  Port=3
  wires:
  Bit Shift/1 -> basic_cycle/1
  Msg_Temporal_Data/1 -> Bit Shift4/1, Bit Shift/1, Bit Shift3/1
  Bit Shift1/1 -> msg_count/1
  Bit Shift2/1 -> board_id/1
  Bit Shift3/1 -> Bit Shift1/1
  Bit Shift4/1 -> Bit Shift2/1

== system HANcoder_E407_TTA_Controller_v3_2/HANcoder STM32 Target - E407-STM32 algorithm/TTA CAN System/TTA System/Matrix Cycle Manager/Backup Board Matrix Cycle/Backup board basic cycle 0/COMP Task - Sync bc0 check/Process_Messages/Demux message CAN1 and check coherence1/msg_count>2_DEBUG ==
  note: If this board received during this COMM a message
      | with a count greater than 1, it means the first message
      | sent was missed, but at least one later msg reached
      | this board.
  msg_c : Inport
  Constant : Constant
  Constant1 : Constant
  Data Store Read : DataStoreRead  DataStoreName=msg_count_DEBUG
  Data Store Read1 : DataStoreRead  DataStoreName=msg_count_DEBUG
  Data Store Write : DataStoreWrite  DataStoreName=msg_count_DEBUG
  GreaterThan : RelationalOperator  Operator=>  OutDataTypeStr=boolean  RndMeth=Simplest
  Plus : Sum
  Switch : Switch  Criteria=u2 > Threshold
  wires:
  msg_c/1 -> GreaterThan/1
  Data Store Read/1 -> Switch/3
  Plus/1 -> Switch/1
  Data Store Read1/1 -> Plus/1
  Constant/1 -> Plus/2
  Switch/1 -> Data Store Write/1
  GreaterThan/1 -> Switch/2
  Constant1/1 -> GreaterThan/2

== system HANcoder_E407_TTA_Controller_v3_2/HANcoder STM32 Target - E407-STM32 algorithm/TTA CAN System/TTA System/Matrix Cycle Manager/Backup Board Matrix Cycle/Backup board basic cycle 1/COMM Task - Sync bc 1/Transmission subtasks1/Check msg transmission CAN1/TX buffer update CAN1 ==
  note: Transmission end - Set message to send through CAN 1
  note: Message Temporal Data
      |    Every message sends
      |    BasicCycle, Tx count
      |    and Verification msg
      |    as data
  note: Transmission ID
      |    Sync Msg: 1
      |    Vote Node 1: 11
      |    Vote Node 2: 12
      |    Vote Node 3: 13
  Tx_ID : Inport
  Msg_Value_Data : Inport  Port=2
  Enable : EnablePort
  Bus Selector : BusSelector  OutputSignals=signal2,signal3,signal4,signal5,signal6,signal7,signal8
  Cast : DataTypeConversion  OutDataTypeStr=uint32
  Cast1 : DataTypeConversion  OutDataTypeStr=uint8
  Cast16 : DataTypeConversion  OutDataTypeStr=uint8
  Cast4 : DataTypeConversion  OutDataTypeStr=uint8
  Data Store Read : DataStoreRead  Priority=50  DataStoreName=Tx_msg_count_CAN1
  Data Store Read1 : DataStoreRead  DataStoreName=Board_ID
  Data Store Read3 : DataStoreRead  DataStoreName=basic_cycle_count
  Data Store Write10 : DataStoreWrite  DataStoreName=Msg_Tx_CAN1  DataStoreElements=Msg_Tx_CAN1.Buffer_1#Msg_Tx_CAN1.Buffer_2#Msg_Tx_CAN1.Buffer_3#Msg_Tx_CAN1.Buffer_4#Msg_Tx_CAN1.Buffer_5#Msg_Tx_CAN1.Buffer_6#Msg_Tx_CAN1.Buffer_7#Msg_Tx_CAN1.Buffer_8
  Data Store Write8 : DataStoreWrite  DataStoreName=TxID_CAN1
  Msg_Data_Encoder : Subsystem
  wires:
  Cast/1 -> Data Store Write8/1
  Data Store Read3/1 -> Cast4/1
  Cast4/1 -> Msg_Data_Encoder/1(basic_cycle)
  Msg_Value_Data/1 -> Bus Selector/1
  Tx_ID/1 -> Cast/1
  Data Store Read/1 -> Cast1/1
  Cast16/1 -> Msg_Data_Encoder/3(board_number)
  Cast1/1 -> Msg_Data_Encoder/2(tx_counter)
  Data Store Read1/1 -> Cast16/1
  Msg_Data_Encoder/1(encoded_msg) -> Data Store Write10/1
  Bus Selector/1 -> Data Store Write10/2  "<signal2>"
  Bus Selector/2 -> Data Store Write10/3  "<signal3>"
  Bus Selector/3 -> Data Store Write10/4  "<signal4>"
  Bus Selector/4 -> Data Store Write10/5  "<signal5>"
  Bus Selector/5 -> Data Store Write10/6  "<signal6>"
  Bus Selector/6 -> Data Store Write10/7  "<signal7>"
  Bus Selector/7 -> Data Store Write10/8  "<signal8>"

== system HANcoder_E407_TTA_Controller_v3_2/HANcoder STM32 Target - E407-STM32 algorithm/TTA CAN System/TTA System/Matrix Cycle Manager/Backup Board Matrix Cycle/Backup board basic cycle 1/COMM Task - Sync bc 1/Transmission subtasks1/Check msg transmission CAN2/TX buffer update CAN2 ==
  note: Transmission end - Set message to send through CAN
  note: Transmission ID
      |    Sync Msg: 1
      |    Vote Node 1: 11
      |    Vote Node 2: 12
      |    Vote Node 3: 13
  note: Message Data
      |    Every message sends
      |    BasicCycle, Tx count
      |    and Verification msg
      |    as data
  Tx_ID : Inport
  Msg_Value_Data : Inport  Port=2
  Enable : EnablePort
  Bus Selector : BusSelector  OutputSignals=signal2,signal3,signal4,signal5,signal6,signal7,signal8
  Cast17 : DataTypeConversion  OutDataTypeStr=uint8
  Cast18 : DataTypeConversion  OutDataTypeStr=uint8
  Cast8 : DataTypeConversion  OutDataTypeStr=uint32
  Cast9 : DataTypeConversion  OutDataTypeStr=uint8
  Data Store Read : DataStoreRead  DataStoreName=Board_ID
  Data Store Read1 : DataStoreRead  Priority=50  DataStoreName=Tx_msg_count_CAN2
  Data Store Read6 : DataStoreRead  DataStoreName=basic_cycle_count
  Data Store Write4 : DataStoreWrite  DataStoreName=Msg_Tx_CAN2  DataStoreElements=Msg_Tx_CAN2.Buffer_1#Msg_Tx_CAN2.Buffer_2#Msg_Tx_CAN2.Buffer_3#Msg_Tx_CAN2.Buffer_4#Msg_Tx_CAN2.Buffer_5#Msg_Tx_CAN2.Buffer_6#Msg_Tx_CAN2.Buffer_7#Msg_Tx_CAN2.Buffer_8
  Data Store Write5 : DataStoreWrite  DataStoreName=TxID_CAN2
  Msg_Data_Encoder : Subsystem
  wires:
  Bus Selector/7 -> Data Store Write4/8  "<signal8>"
  Bus Selector/6 -> Data Store Write4/7  "<signal7>"
  Bus Selector/5 -> Data Store Write4/6  "<signal6>"
  Bus Selector/4 -> Data Store Write4/5  "<signal5>"
  Bus Selector/3 -> Data Store Write4/4  "<signal4>"
  Bus Selector/2 -> Data Store Write4/3  "<signal3>"
  Bus Selector/1 -> Data Store Write4/2  "<signal2>"
  Msg_Value_Data/1 -> Bus Selector/1
  Data Store Read/1 -> Cast17/1
  Cast8/1 -> Data Store Write5/1
  Cast9/1 -> Msg_Data_Encoder/2(tx_counter)
  Tx_ID/1 -> Cast8/1
  Cast17/1 -> Msg_Data_Encoder/3(verif_value)
  Data Store Read6/1 -> Cast18/1
  Msg_Data_Encoder/1(encoded_msg) -> Data Store Write4/1
  Data Store Read1/1 -> Cast9/1
  Cast18/1 -> Msg_Data_Encoder/1(basic_cycle)

== system HANcoder_E407_TTA_Controller_v3_2/HANcoder STM32 Target - E407-STM32 algorithm/TTA CAN System/TTA System/Matrix Cycle Manager/Backup Board Matrix Cycle/Backup board basic cycle 1/COMM Task - Sync bc 1/Transmission subtasks1/Msg_Value_Data_Encoded/float2uint1 ==
  precision : Inport
  magnitude : Inport  Port=2
  magnitude_max : Inport  Port=3
  magnitude_min : Inport  Port=4
  Abs : Abs
  Bit Shift : hdlsllib/Logic and Bit Operations/Bit Shift  mode=Shift Left Logical  N=7
      settings: SourceProductName=HDL Coder  SourceProductBaseCode=HD
  Cast : DataTypeConversion  OutDataTypeStr=uint8
  Cast1 : DataTypeConversion  OutDataTypeStr=uint8
  Cast2 : DataTypeConversion  OutDataTypeStr=uint8
  Constant : Constant  Value=0
  Constant1 : Constant  Value=2
  Constant2 : Constant  Value=2
  Divide : Product  Inputs=*/
  Fix : Rounding  Priority=3  Operator=fix
  Fix1 : Rounding  Priority=6  Operator=fix
  Gain : Gain  Gain=-1
  GreaterThan : RelationalOperator  Priority=2  Operator=<  OutDataTypeStr=boolean  RndMeth=Simplest
  LessThanOrEqual1 : RelationalOperator  OutDataTypeStr=boolean  RndMeth=Simplest
  LessThanOrEqual2 : RelationalOperator  Operator=<  OutDataTypeStr=boolean  RndMeth=Simplest
  Minus : Sum  Priority=4  Inputs=-+
  Multiply : Product
  Plus : Sum  Priority=10  Inputs=+++
  Power : Math  Priority=5  Operator=pow  SaturateOnIntegerOverflow=on
  Power1 : Math  Priority=5  Operator=pow  SaturateOnIntegerOverflow=on
  Switch : Switch  Criteria=u2 > Threshold
  Switch1 : Switch  Criteria=u2 > Threshold
  Switch2 : Switch  Criteria=u2 > Threshold
  coded : Outport
  wires:
  Switch1/1 -> Switch2/3
  Switch/1 -> Switch2/1
  LessThanOrEqual1/1 -> Switch1/2
  LessThanOrEqual2/1 -> Switch/2, Switch2/2
  magnitude_max/1 -> LessThanOrEqual2/1, Switch/1
  magnitude_min/1 -> Switch1/3, LessThanOrEqual1/2
  magnitude/1 -> Switch/3, LessThanOrEqual2/2, Switch1/1, LessThanOrEqual1/1
  Plus/1 -> coded/1
  [prec] -> Power1/2
  Multiply/1 -> Cast1/1
  precision/1 -> Gain/1, [prec]
  Power1/1 -> Multiply/2
  Constant2/1 -> Power1/1
  Cast2/1 -> Plus/3
  Fix1/1 -> Cast2/1
  Divide/1 -> Fix1/1
  Power/1 -> Divide/2
  Gain/1 -> Power/2
  Constant1/1 -> Power/1
  Cast1/1 -> Plus/2
  Bit Shift/1 -> Plus/1
  Cast/1 -> Bit Shift/1
  Minus/1 -> Divide/1
  Fix/1 -> Minus/1, Multiply/1
  GreaterThan/1 -> Cast/1
  Abs/1 -> Fix/1, Minus/2
  Switch2/1 -> GreaterThan/1, Abs/1
  Constant/1 -> GreaterThan/2
